simulink model "SG__MDL"  (R2022b)
settings: Solver=FixedStepAuto  StartTime=0.0  StopTime=Inf  FixedStep=5e-05  RelTol=1e-3  EnableMultiTasking=on
model workspace (MAT data in the model file):
  Bl = Simulink.Parameter
  Bl.Value = [1.7294 2.4096]
  Bl.Description = 'current to voltage conversion'
  Bl.DataType = 'auto'
  Bl.Complexity = 'real'
  Bl.Dimensions = [1 2]
  Csb = Simulink.Parameter
  Csb.Value = [1e-06 1e-06]
  Csb.DataType = 'auto'
  Csb.Complexity = 'real'
  Csb.Dimensions = [1 2]
  N_trig = Simulink.Parameter
  N_trig.Value = 32
  N_trig.Description = 'number of samples for triggered pulse for recording'
  N_trig.DataType = 'uint32'
  N_trig.Complexity = 'real'
  N_trig.Dimensions = [1 1]
  Sd = Simulink.Parameter
  Sd.Value = 0.0032
  Sd.Description = 'current to voltage conversion'
  Sd.DataType = 'auto'
  Sd.Complexity = 'real'
  Sd.Dimensions = [1 1]
  alpha_mat = Simulink.Parameter
  alpha_mat.Value = [1  1  1; 1  1  1]
  alpha_mat.DataType = 'auto'
  alpha_mat.Complexity = 'real'
  alpha_mat.Dimensions = [2 3]
  beta_mat = Simulink.Parameter
  beta_mat.Value = [0.5  0.5  0.5; 0.5  0.5  0.5]
  beta_mat.DataType = 'auto'
  beta_mat.Complexity = 'real'
  beta_mat.Dimensions = [2 3]
  dtf_a = Simulink.Parameter
  dtf_a.Value = [1  1  1; 1  1  1]
  dtf_a.DataType = 'auto'
  dtf_a.Complexity = 'real'
  dtf_a.Dimensions = [2 3]
  dtf_b = Simulink.Parameter
  dtf_b.Value = [0.5  0.5  0.5; 0.5  0.5  0.5]
  dtf_b.DataType = 'auto'
  dtf_b.Complexity = 'real'
  dtf_b.Dimensions = [2 3]
  enable_source = Simulink.Parameter
  enable_source.Value = 0
  enable_source.DataType = 'boolean'
  enable_source.Complexity = 'real'
  enable_source.Dimensions = [1 1]
  freq_0 = Simulink.Parameter
  freq_0.Value = 602
  freq_0.Description = 'tube fundamental resonance frequency
    | '
  freq_0.DataType = 'auto'
  freq_0.Complexity = 'real'
  freq_0.Dimensions = [1 1]
  harm_corr = Simulink.Parameter
  harm_corr.Value = [1; 1]
  harm_corr.DataType = 'auto'
  harm_corr.Complexity = 'real'
  harm_corr.Dimensions = [2 1]
  i2u = Simulink.Parameter
  i2u.Value = 100
  i2u.Description = 'current to voltage conversion'
  i2u.DataType = 'auto'
  i2u.Complexity = 'real'
  i2u.Dimensions = [1 1]
  omega_0_vec = Simulink.Parameter
  omega_0_vec.Value = [2000 2000]
  omega_0_vec.DataType = 'auto'
  omega_0_vec.Complexity = 'real'
  omega_0_vec.Dimensions = [1 2]
  phi = Simulink.Parameter
  phi.Value = [0; 0]
  phi.DataType = 'auto'
  phi.Complexity = 'real'
  phi.Dimensions = [2 1]
  rec = Simulink.Parameter
  rec.Value = 0
  rec.DataType = 'boolean'
  rec.Complexity = 'real'
  rec.Dimensions = [1 1]
  rho = Simulink.Parameter
  rho.Value = [1; 1]
  rho.DataType = 'auto'
  rho.Complexity = 'real'
  rho.Dimensions = [2 1]
  rho_corr = Simulink.Parameter
  rho_corr.Value = [1; 1]
  rho_corr.DataType = 'auto'
  rho_corr.Complexity = 'real'
  rho_corr.Dimensions = [2 1]
  sens_p = Simulink.Parameter
  sens_p.Value = [0; 0; 0; 0]
  sens_p.DataType = 'auto'
  sens_p.Complexity = 'real'
  sens_p.Dimensions = [4 1]
  src_gain = Simulink.Parameter
  src_gain.Value = 0.005
  src_gain.DataType = 'auto'
  src_gain.Complexity = 'real'
  src_gain.Dimensions = [1 1]
  theta = Simulink.Parameter
  theta.Value = [3.14159265359; 0]
  theta.DataType = 'auto'
  theta.Complexity = 'real'
  theta.Dimensions = [2 1]
  ts_ctr = Simulink.Parameter
  ts_ctr.Value = 5e-05
  ts_ctr.DataType = 'auto'
  ts_ctr.Complexity = 'real'
  ts_ctr.Dimensions = [1 1]
libraries: simulink x4, speedgoatlib_IO135 x3, hdlsllib x2, slrealtimeloglib x1, dspsigops x1
settings Model: SimulationMode=external  ExtModeEnableFloating=off  DataflowThreadingImplementation=Pthreads  Creator=padlewsk  LastModifiedBy=padlewsk
settings SolverCC: ConcurrentTasks=on  AlgebraicLoopSolver=TrustRegion  PositivePriorityOrder=on  AutoInsertRateTranBlk=on
settings DataIOCC: SaveFormat=StructureWithTime
settings OptimizationCC: DefaultParameterBehavior=Inlined  GainParamInheritBuiltInType=on  UseFloatMulNetSlope=on  RollThreshold=9  EfficientFloat2IntCast=on  SimCompilerOptimization=on
settings DebuggingCC: ReadBeforeWriteMsg=DisableAll  WriteAfterWriteMsg=DisableAll  WriteAfterReadMsg=DisableAll  TasksWithSamePriorityMsg=none  UnconnectedInputMsg=warning  UnconnectedOutputMsg=warning  UnconnectedLineMsg=warning  ModelReferenceSymbolNameMessage=none
settings HardwareCC: ProdBitPerLong=64  ProdLongLongMode=on  ProdHWDeviceType=Intel->x86-64 (Linux 64)
settings ModelReferenceCC: UpdateModelReferenceTargets=IfOutOfDate  EnableRefExpFcnMdlSchedulingChecks=on
settings SFSimCC: SFSimEcho=off
settings RTWCC: Description=Simulink Real-Time  SystemTargetFile=slrealtime.tlc  TemplateMakefile=slrealtime_default_tmf  Toolchain=Simulink Real-Time Toolchain  BuildConfiguration=Faster Runs  CodeExecutionProfiling=on  TargetLang=C++
settings SimulinkRealTimeTargetCC: UseGCCFastMath=on

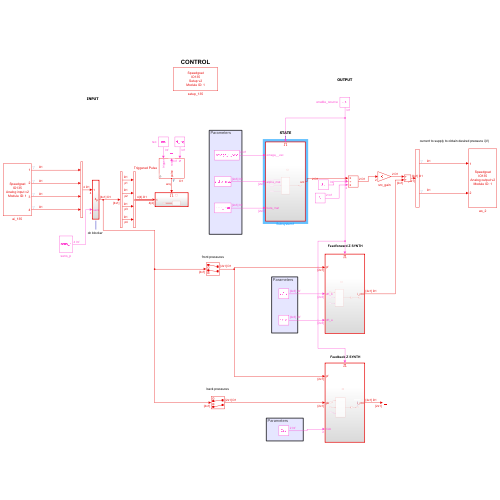
[thumbnail: Simulink's stored preview of the top-level diagram]
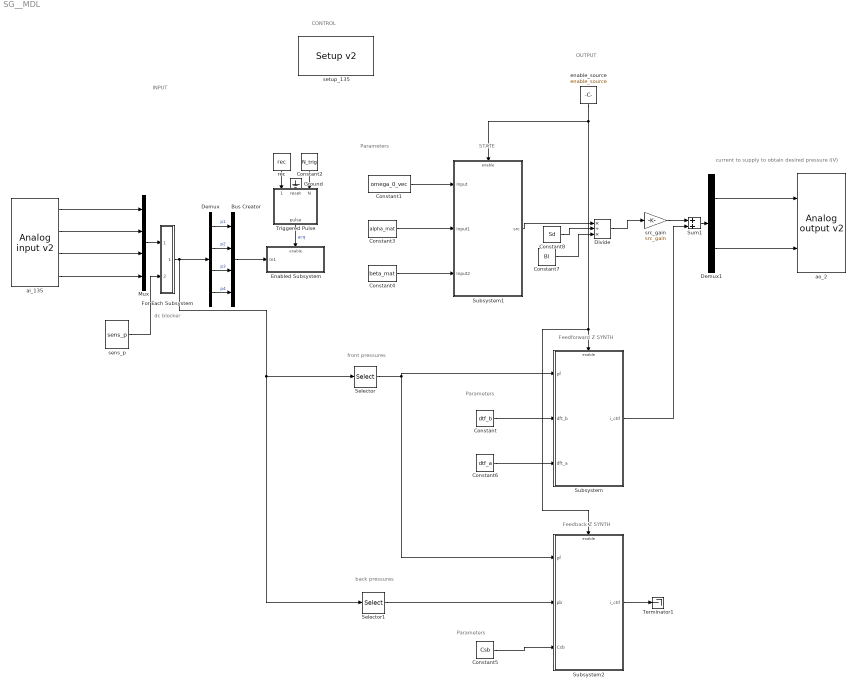
== system SG__MDL ==
  note: Parameters
  note: front pressures
  note: dc blocker
  note: Parameters
  note: CONTROL
  note: INPUT
  note: OUTPUT
  note: current to supply to obtain desired pressure i(V)
  note: Parameters
  note: STATE
  note: Feedforward Z SYNTH
  note: Feedback Z SYNTH
  note: back pressures
  Bus Creator : BusCreator  Inputs=4
  Constant : Constant  Value=dtf_b
  Constant1 : Constant  Value=omega_0_vec
  Constant2 : Constant  Value=N_trig
  Constant3 : Constant  Value=alpha_mat
  Constant4 : Constant  Value=beta_mat
  Constant5 : Constant  Value=Csb
  Constant6 : Constant  Value=dtf_a
  Constant7 : Constant  Value=Bl
  Constant8 : Constant  Value=Sd
  Demux : Demux
  Demux1 : Demux  Outputs=2
  Divide : Product  Inputs=*/*
  Enabled Subsystem : Subsystem  TreatAsAtomicUnit=on
  For Each Subsystem : Subsystem  TreatAsAtomicUnit=on
  Ground : Ground
  Mux : Mux
  Selector : Selector  InputPortWidth=4  IndexOptions=Index vector (dialog)  Indices=[1 3]  OutputSizes=1
  Selector1 : Selector  InputPortWidth=4  IndexOptions=Index vector (dialog)  Indices=[2 4]  OutputSizes=1
  Subsystem : Subsystem
  Subsystem1 : Subsystem
  Subsystem2 : Subsystem
  Sum1 : Sum
  Terminator1 : Terminator
  Triggered Pulse : Subsystem  mask(Triggered Pulse){}
      mask help: Generates a single pulse of N samples length
  ai_135 : speedgoatlib_IO135/Analog input v2   parModuleId=1  parSampleTime=-1  parPciSlot=-1  parAdcChannels=[1 2 3 4]  parAdcVoltageRange=[1 1 1 1]  parAdcOversamplRate=[1 1 1 1]  parAdcContSampling=0  parAdcDmaEnable=0  parAdcActiveDmaDevices=[1 1 1 1]  parAdcFrameSize=1
      settings: SourceProductName=Simulink Real-Time: Speedgoat I/O Blockset
  ao_2 : speedgoatlib_IO135/Analog output v2   parModuleId=1  parSampleTime=-1  parPciSlot=-1  parDacChannels=[1 2]  parDacVoltageRange=[5 5 4 4 4 4 4 4 4 4 4 4 4 4 4 4]  parDacInitValues=[0 0]  parDacReset=[1 1]  parDacSyncOut=1  parDacDmaEnable=0  parDacActiveDmaDevices=[1 1 1 1]  parDacDmaLatency=1  parDacFrameSize=1
      settings: SourceProductName=Simulink Real-Time: Speedgoat I/O Blockset
  enable_source : Constant  Value=enable_source
  rec : Constant  Value=rec
  sens_p : Constant  Value=sens_p
  setup_135 : speedgoatlib_IO135/Setup v2   parPciSlot=-1  parModuleId=1  parInterModuleSync=None  parConvClockBaseRate=20MHz  parConvClock1Divider=700  parConvClock2Divider=700  parFrameTriggerEnable=off  parFrameTriggerDivider=10  parConvClock1BaseRate=1  parConvClock2BaseRate=1  parFrameTriggerClock=1  parAdcChannels=[1:4]  parAdcRange1=+-5V  parAdcRange2=+-5V  parAdcRange3=+-5V  parAdcRange4=+-5V  parAdcVoltageRange=[1 1 1 1]  parAdcOversampling1=None  parAdcOversampling2=None  parAdcOversampling3=None  parAdcOversampling4=None  parAdcOversamplRate=[1 1 1 1]  parAdcAutoCorrection=on  parAdcContSampling=off  parAdcDmaEnable=off  parAdcDmaClock=Clock 1  parAdcFrameSize_=1  parAdcSampleTime_=-1  parAdcActiveDmaDevices=[1 1 1 1]  parAdcFrameTriggerEnable=0  parAdcFrameSize=1  parAdcSampleTime=3.5e-05  parDacChannels=[1:2]  parDacInitValues=zeros(1,2)  parDacReset=1  parDacRange1=+-10V  parDacRange2=+-10V  parDacRange3=+-5V  parDacRange4=+-5V  parDacRange5=+-5V  parDacRange6=+-5V  parDacRange7=+-5V  parDacRange8=+-5V  parDacRange9=+-5V  parDacRange10=+-5V  parDacRange11=+-5V  parDacRange12=+-5V  parDacRange13=+-5V  parDacRange14=+-5V  parDacRange15=+-5V  parDacRange16=+-5V  parDacVoltageRange=[5 5 4 4 4 4 4 4 4 4 4 4 4 4 4 4]  parDacAutoCorrection=on  parDacSyncOut=on  parDacDmaEnable=off  parDacDmaLatency=As small as possible  parDacDmaClock=Clock 1  parDacFrameSize_=1  parDacSampleTime_=-1  parDacActiveDmaDevices=[1 1 1 1]  parDacFrameTriggerEnable=0  parDacFrameSize=1  parDacSampleTime=3.5e-05  parDoChannels=[]  parDoInitValues=0  parDoReset=1  parDiChannels=[]  parDiDebounceEnable=off  parDiDebounceTime=0  parDiDebounceValue=0  parDioPullRefFront=Pull-up 3.3V  parDioPullRefRear=Floating
      settings: SourceProductName=Simulink Real-Time: Speedgoat I/O Blockset
  src_gain : Gain  Gain=src_gain
  wires:
  ai_135/2 -> Mux/2
  ai_135/1 -> Mux/1
  Mux/1 -> For Each Subsystem/1(In1)
  For Each Subsystem/1(p) -> Selector1/1, Selector/1, Demux/1
  Bus Creator/1 -> Enabled Subsystem/1(In1)
  Demux/1 -> Bus Creator/1  "p1"
  Demux/2 -> Bus Creator/2  "p2"
  Triggered Pulse/1(pulse) -> Enabled Subsystem/Enable  "acq"
  Ground/1 -> Triggered Pulse/2(reset)
  rec/1 -> Triggered Pulse/1(trigger)
  Constant2/1 -> Triggered Pulse/3(N)
  sens_p/1 -> For Each Subsystem/2(sens_p)
  Constant/1 -> Subsystem/2(dft_b)
  Constant6/1 -> Subsystem/3(dft_a)
  enable_source/1 -> Subsystem2/Enable, Subsystem/Enable, Subsystem1/Enable
  ai_135/3 -> Mux/3
  ai_135/4 -> Mux/4
  Demux/3 -> Bus Creator/3  "p3"
  Demux/4 -> Bus Creator/4  "p4"
  Constant4/1 -> Subsystem1/3(Input2)
  Constant3/1 -> Subsystem1/2(Input1)
  Constant1/1 -> Subsystem1/1(Input)
  Demux1/1 -> ao_2/1
  Constant5/1 -> Subsystem2/3(Csb)
  Subsystem2/1(i_ctrl) -> Terminator1/1
  Selector1/1 -> Subsystem2/2(pb)
  Demux1/2 -> ao_2/2
  Selector/1 -> Subsystem/1(pf), Subsystem2/1(pf)
  Subsystem/1(i_ctrl) -> Sum1/2
  Sum1/1 -> Demux1/1
  src_gain/1 -> Sum1/1
  Subsystem1/1(src) -> Divide/1
  Divide/1 -> src_gain/1
  Constant7/1 -> Divide/3
  Constant8/1 -> Divide/2

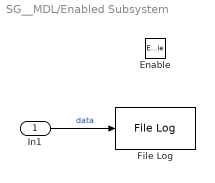
== system SG__MDL/Enabled Subsystem ==
  In1 : Inport
  Enable : EnablePort
  File Log : slrealtimeloglib/File Log  decimation=1  inputProcessing=Elements as channels (sample based)
  wires:
  In1/1 -> File Log/1  "data"

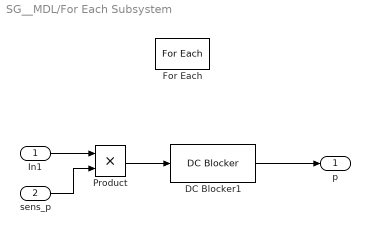
== system SG__MDL/For Each Subsystem ==
  In1 : Inport  Partition=on  PartitionDimension=1  PartitionWidth=1  PartitionOffset=0
  sens_p : Inport  Port=2  Partition=on  PartitionDimension=1  PartitionWidth=1  PartitionOffset=0
  DC Blocker1 : dspsigops/DC Blocker  Algorithm=IIR  NormalizedBandwidth=0.001  Length=50  Order=3  SimulateUsing=Code generation
      settings: LibrarySourceBlock=dsphdlsupportsigops/DC Blocker
  For Each : ForEach  DisableCoverage=on
  Product : Product
  p : Outport  ConcatenationDimension=1
  wires:
  sens_p/1 -> Product/2
  Product/1 -> DC Blocker1/1
  DC Blocker1/1 -> p/1
  In1/1 -> Product/1

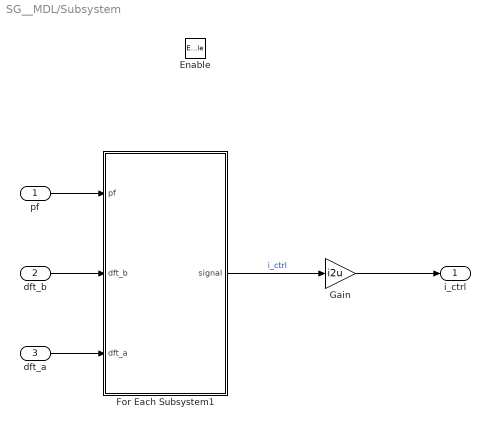
== system SG__MDL/Subsystem ==
  pf : Inport
  dft_b : Inport  Port=2
  dft_a : Inport  Port=3
  Enable : EnablePort
  For Each Subsystem1 : Subsystem  TreatAsAtomicUnit=on
  Gain : Gain  Gain=i2u
  i_ctrl : Outport
  wires:
  pf/1 -> For Each Subsystem1/1(pf)
  dft_b/1 -> For Each Subsystem1/2(dft_b)
  For Each Subsystem1/1(signal) -> Gain/1  "i_ctrl"
  dft_a/1 -> For Each Subsystem1/3(dft_a)
  Gain/1 -> i_ctrl/1

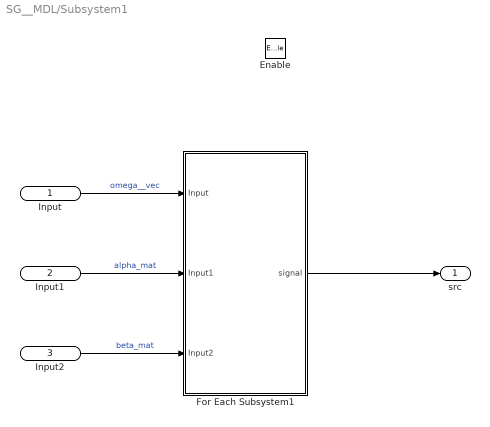
== system SG__MDL/Subsystem1 ==
  Input : Inport
  Input1 : Inport  Port=2
  Input2 : Inport  Port=3
  Enable : EnablePort
  For Each Subsystem1 : Subsystem  TreatAsAtomicUnit=on
  src : Outport
  wires:
  For Each Subsystem1/1(signal) -> src/1
  Input/1 -> For Each Subsystem1/1(Input)  "omega__vec"
  Input1/1 -> For Each Subsystem1/2(Input1)  "alpha_mat"
  Input2/1 -> For Each Subsystem1/3(Input2)  "beta_mat"

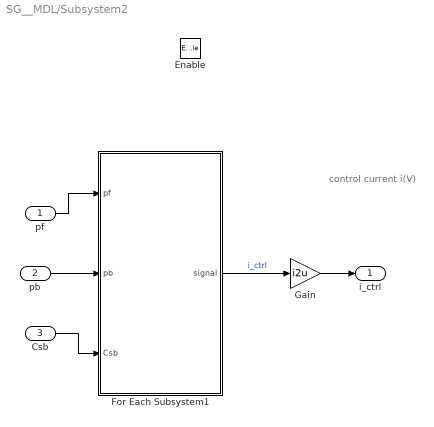
== system SG__MDL/Subsystem2 ==
  note: control current i(V)
  pf : Inport
  pb : Inport  Port=2
  Csb : Inport  Port=3
  Enable : EnablePort
  For Each Subsystem1 : Subsystem  TreatAsAtomicUnit=on
  Gain : Gain  Gain=i2u
  i_ctrl : Outport
  wires:
  pf/1 -> For Each Subsystem1/1(pf)
  For Each Subsystem1/1(signal) -> Gain/1  "i_ctrl"
  Csb/1 -> For Each Subsystem1/3(Csb)
  pb/1 -> For Each Subsystem1/2(pb)
  Gain/1 -> i_ctrl/1

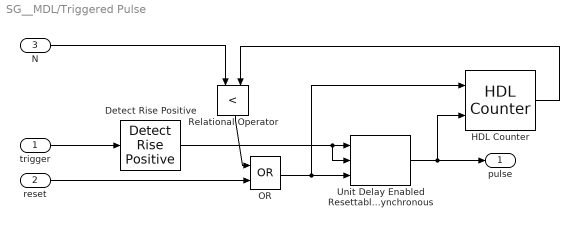
== system SG__MDL/Triggered Pulse ==
  trigger : Inport
  reset : Inport  Port=2
  N : Inport  Port=3
  Detect Rise Positive : simulink/Logic and Bit Operations/Detect Rise Positive  vinit=0  OutDataTypeStr=boolean
  HDL Counter : hdlsllib/Sources/HDL Counter  CountType=Free running  CountInit=1  CountStep=1  CountMax=25  CountFromType=Initial value  CountFrom=1  CountResetPort=on  CountLoadPort=off  CountEnbPort=on  CountDirPort=off  CountHitOutputPort=off  CountDataType=Unsigned  CountWordLen=32  CountFracLen=0  CountSampTime=1
  OR : Logic  Operator=OR  AllPortsSameDT=off  OutDataTypeStr=boolean
  Relational Operator : RelationalOperator  Operator=<  OutDataTypeStr=boolean  RndMeth=Simplest  InputSameDT=off
  Unit Delay Enabled Resettable Synchronous : hdlsllib/Discrete/Unit Delay Enabled Resettable Synchronous  InitialCondition=0.0  SampleTime=-1
  pulse : Outport  VectorParamsAs1DForOutWhenUnconnected=off
  wires:
  N/1 -> Relational Operator/1
  HDL Counter/1 -> Relational Operator/2
  Detect Rise Positive/1 -> Unit Delay Enabled Resettable Synchronous/2, Unit Delay Enabled Resettable Synchronous/1
  reset/1 -> OR/2
  Relational Operator/1 -> OR/1
  Unit Delay Enabled Resettable Synchronous/1 -> pulse/1, HDL Counter/2
  trigger/1 -> Detect Rise Positive/1
  OR/1 -> HDL Counter/1, Unit Delay Enabled Resettable Synchronous/3

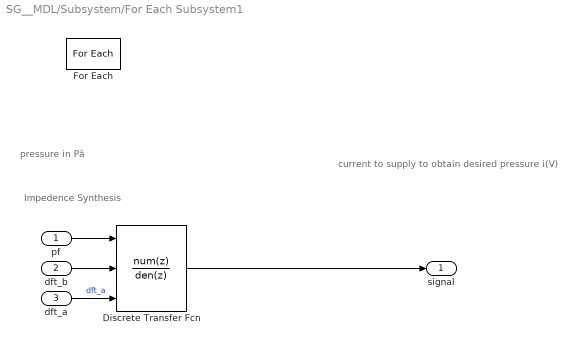
== system SG__MDL/Subsystem/For Each Subsystem1 ==
  note: pressure in Pâ
  note: Impedence Synthesis
  note: current to supply to obtain desired pressure i(V)
  pf : Inport  Partition=on  PartitionDimension=1  PartitionWidth=1  PartitionOffset=0
  dft_b : Inport  Port=2  Partition=on  PartitionDimension=1  PartitionWidth=1  PartitionOffset=0
  dft_a : Inport  Port=3  Partition=on  PartitionDimension=1  PartitionWidth=1  PartitionOffset=0
  Discrete Transfer Fcn : DiscreteTransferFcn  NumeratorSource=Input port  DenominatorSource=Input port  a0EqualsOne=on
      settings: InputPortMap=u0,p1,p3
  For Each : ForEach  DisableCoverage=on
  signal : Outport  OutputWhenDisabled=reset  InitialOutput=0  ConcatenationDimension=1  VectorParamsAs1DForOutWhenUnconnected=off
  wires:
  dft_b/1 -> Discrete Transfer Fcn/2
  dft_a/1 -> Discrete Transfer Fcn/3  "dft_a"
  Discrete Transfer Fcn/1 -> signal/1
  pf/1 -> Discrete Transfer Fcn/1

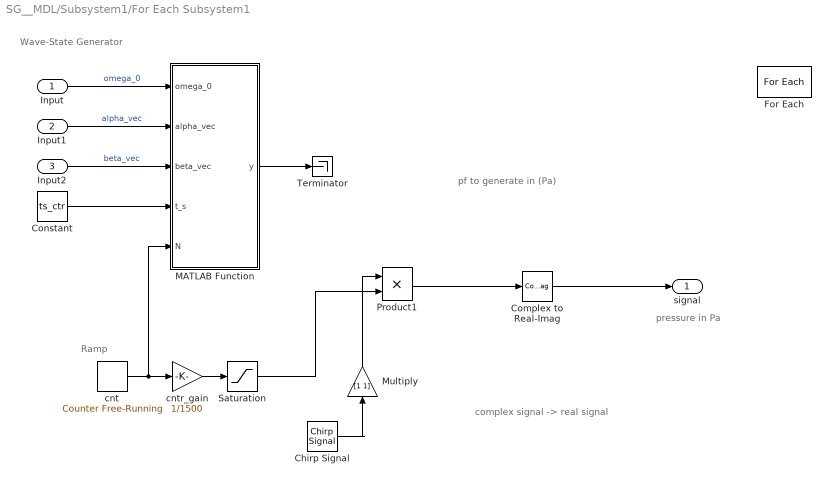
== system SG__MDL/Subsystem1/For Each Subsystem1 ==
  note: pressure in Pa
  note: pf to generate in (Pa)
  note: Wave-State Generator
  note: Ramp
  note: complex signal -> real signal
  Input : Inport  Partition=on  PartitionDimension=1  PartitionWidth=1  PartitionOffset=0
  Input1 : Inport  Port=2  Partition=on  PartitionDimension=1  PartitionWidth=1  PartitionOffset=0
  Input2 : Inport  Port=3  Partition=on  PartitionDimension=1  PartitionWidth=1  PartitionOffset=0
  Chirp Signal : simulink/Sources/Chirp Signal  f1=10  T=5  f2=1000
  Complex to Real-Imag : ComplexToRealImag  Output=Real
  Constant : Constant  Value=ts_ctr  SampleTime=-1
  For Each : ForEach  DisableCoverage=on
  MATLAB Function : MATLAB Function  TreatAsAtomicUnit=on
  Multiply : Gain  Gain=[1 1]
  Product1 : Product
  Saturation : Saturate  UpperLimit=1  LowerLimit=0
  Terminator : Terminator
  cnt : simulink/Sources/Counter Free-Running  NumBits=32  tsamp=-1
  cntr_gain : Gain  Gain=1/1500  ParamDataTypeStr=double
  signal : Outport  OutputWhenDisabled=reset  InitialOutput=0  ConcatenationDimension=1  VectorParamsAs1DForOutWhenUnconnected=off
  wires:
  cnt/1 -> MATLAB Function/5(N), cntr_gain/1
  Saturation/1 -> Product1/2
  cntr_gain/1 -> Saturation/1
  Constant/1 -> MATLAB Function/4(t_s)
  Product1/1 -> Complex to Real-Imag/1
  Complex to Real-Imag/1 -> signal/1
  Input/1 -> MATLAB Function/1(omega_0)  "omega_0"
  Input1/1 -> MATLAB Function/2(alpha_vec)  "alpha_vec"
  Input2/1 -> MATLAB Function/3(beta_vec)  "beta_vec"
  MATLAB Function/1(y) -> Terminator/1
  Chirp Signal/1 -> Multiply/1
  Multiply/1 -> Product1/1

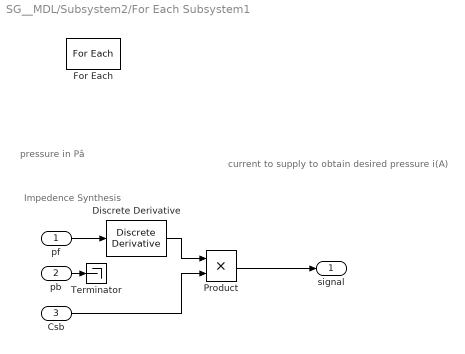
== system SG__MDL/Subsystem2/For Each Subsystem1 ==
  note: pressure in Pâ
  note: Impedence Synthesis
  note: current to supply to obtain desired pressure i(A)
  pf : Inport  Partition=on  PartitionDimension=1  PartitionWidth=1  PartitionOffset=0
  pb : Inport  Port=2  Partition=on  PartitionDimension=1  PartitionWidth=1  PartitionOffset=0
  Csb : Inport  Port=3  Partition=on  PartitionDimension=1  PartitionWidth=1  PartitionOffset=0
  Discrete Derivative : simulink/Discrete/Discrete Derivative  gainval=1.0  ICPrevScaledInput=0.0  OutMin=[]  OutMax=[]  OutDataType=fixdt(1, 16)  OutScaling=2^-10  DoSatur=off
  For Each : ForEach  DisableCoverage=on
  Product : Product
  Terminator : Terminator
  signal : Outport  OutputWhenDisabled=reset  InitialOutput=0  ConcatenationDimension=1  VectorParamsAs1DForOutWhenUnconnected=off
  wires:
  Csb/1 -> Product/2
  Product/1 -> signal/1
  pf/1 -> Discrete Derivative/1
  Discrete Derivative/1 -> Product/1
  pb/1 -> Terminator/1

== matlab function SG__MDL/Subsystem1/For Each Subsystem1/MATLAB Function ==
  data: omega_0 input; y output; alpha_vec input; beta_vec input; t_s input; N input
function y = fcn(omega_0, alpha_vec, beta_vec, t_s,N) % gamma_vec = [gamma_0, gamma_1,gamma_2....] harm_corr? rho_corr?
    omega_1 = 2*omega_0; % orthogonal state representations
    t = double(N)*t_s;
    
    % Define Quantum Entanglement Channels
    Omega = 8*omega_0; % 1st quantum entanglement channel
    Omega_vec = Omega*[0:(length(alpha_vec)-1)]'; % harmonics of the 1QEC starting with DC channel (see __20241104__)

    alpha_t = alpha_vec*exp(1i*Omega_vec*t);
    beta_t  =  beta_vec*exp(1i*Omega_vec*t);

    psi =  alpha_t*exp(-1i*omega_0*t) + beta_t*exp(-1i*omega_1*t);
    y = psi;
end
